simulink model "Sine_Saturation_Block"  (R2022a)
settings: Solver=VariableStepAuto  StartTime=0.0  StopTime=20  RelTol=1e-3
undefined symbols (not defined in the file or in its folder): canChannel
libraries: canlib x4, canmsglib x2
settings Model: Creator=maxju  LastModifiedBy=maxju

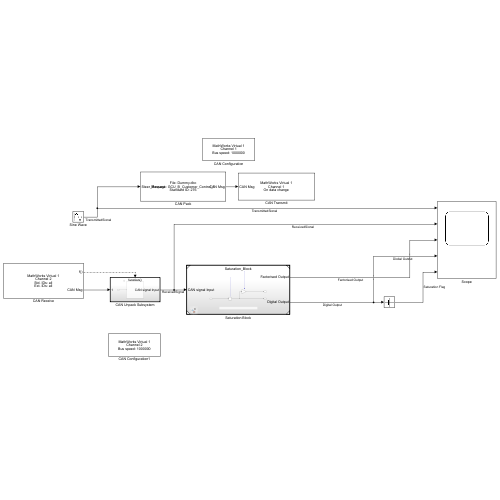
[thumbnail: Simulink's stored preview of the top-level diagram]
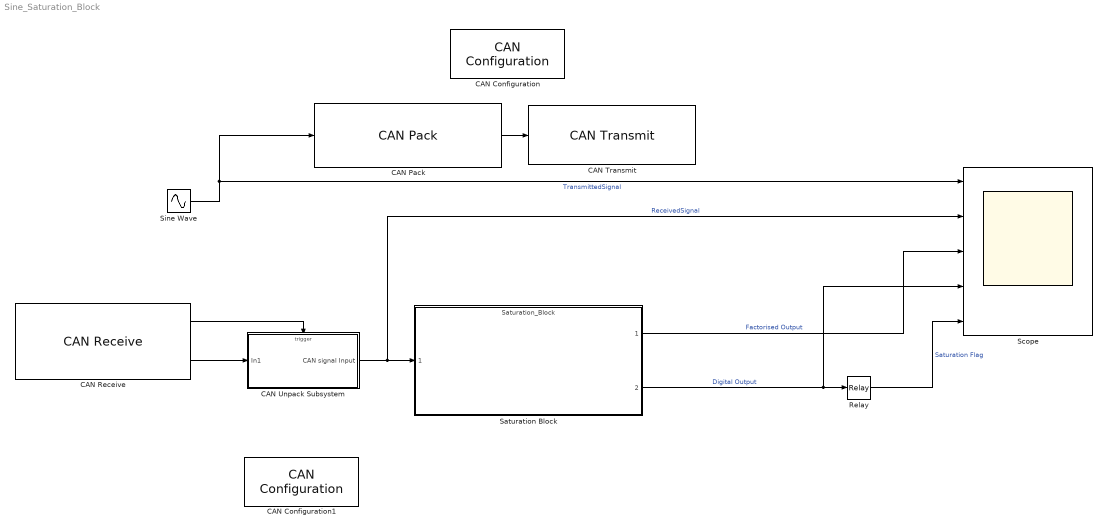
== system Sine_Saturation_Block ==
  CAN Configuration : canlib/CAN Configuration  BlockHandle=2.0009  Device=MathWorks Virtual 1 (Channel 1)  DeviceMenu=MathWorks Virtual 1 (Channel 1)  ObjConstructor=canChannel('MathWorks', 'Virtual 1', 1)  BusSpeed=1000000  EnableBitParameters=off  AckMode=Normal
      settings: SourceProductBaseCode=VN
  CAN Configuration1 : canlib/CAN Configuration  BlockHandle=3.0004  Device=MathWorks Virtual 1 (Channel 2)  DeviceMenu=MathWorks Virtual 1 (Channel 2)  ObjConstructor=canChannel('MathWorks', 'Virtual 1', 2)  BusSpeed=1000000  EnableBitParameters=off  AckMode=Normal
      settings: SourceProductBaseCode=VN
  CAN Pack : canmsglib/CAN Pack  CANdbFile=C:\Workspace\SIMULINK-Models\CAN_Saturation_Block\Dummy.dbc  MsgList=GCU_B_Customer_Control_1  MsgName=GCU_B_Customer_Control_1  MsgIDType=Standard (11-bit identifier)  MsgIdentifier=276  MsgLength=8  Remote=off  ApplyMinMax=off  BusOutput=off  SignalInfo={'Steer_Request','56','64','BE','signed','Standard','0','1','0','-100','100'}
      settings: SourceProductBaseCode=XP,ME,VN  DataFormat=CANdb specified signals
  CAN Receive : canlib/CAN Receive  BlockHandle=7.0004  Device=MathWorks Virtual 1 (Channel 2)  DeviceMenu=MathWorks Virtual 1 (Channel 2)  ObjConstructor=canChannel('MathWorks', 'Virtual 1', 2)  EnableStandardIDsFilter=off  StdIDsCombo=Allow all  StandardIDs=0  EnableExtendedIDsFilter=off  ExtIDsCombo=Allow all  ExtendedIDs=0  SampleTime=0.01  MsgsPerTimestep=1  InternalFilterUpdateStatus=on  BusOutput=off
      settings: SourceProductBaseCode=VN
  CAN Transmit : canlib/CAN Transmit  BlockHandle=10.0004  Device=MathWorks Virtual 1 (Channel 1)  DeviceMenu=MathWorks Virtual 1 (Channel 1)  ObjConstructor=canChannel('MathWorks', 'Virtual 1', 1)  EnableEventTransmit=on  EnablePeriodicTransmit=off  MessagePeriod=1.000
      settings: SourceProductBaseCode=VN
  CAN Unpack Subsystem : Subsystem  TreatAsAtomicUnit=on
  Relay : Relay  OnSwitchValue=[100 -100]  OffSwitchValue=[100 -100]  OnOutputValue=130
  Saturation Block : ModelReference  ModelNameDialog=Saturation_Block.slx  SimulationMode=Normal  ModelReferenceVersion=1.5
  Scope : Scope  NumInputPorts=5
  Sine Wave : Sin  SineType=Sample based  Amplitude=114  Samples=100  SampleTime=0.01
  wires:
  CAN Pack/1 -> CAN Transmit/1
  Sine Wave/1 -> CAN Pack/1, Scope/1  "TransmittedSignal"
  CAN Receive/2 -> CAN Unpack Subsystem/1(In1)
  CAN Receive/1 -> CAN Unpack Subsystem/Trigger
  Saturation Block/1 -> Scope/3  "Factorised Output"
  Saturation Block/2 -> Relay/1, Scope/4  "Digital Output"
  CAN Unpack Subsystem/1(CAN signal Input) -> Scope/2, Saturation Block/1  "ReceivedSignal"
  Relay/1 -> Scope/5  "Saturation Flag"

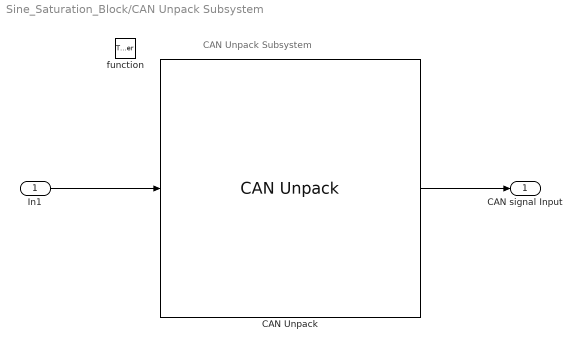
== system Sine_Saturation_Block/CAN Unpack Subsystem ==
  note: CAN Unpack Subsystem
  In1 : Inport
  function : TriggerPort  TriggerType=function-call  VariantControl=Variant
  CAN Unpack : canmsglib/CAN Unpack  CANdbFile=C:\Workspace\SIMULINK-Models\CAN_Saturation_Block\Dummy.dbc  MsgList=GCU_B_Customer_Control_1  MsgName=GCU_B_Customer_Control_1  MsgIDType=Standard (11-bit identifier)  MsgIdentifier=276  MsgLength=8  SignalInfo={'Steer_Request','56','64','BE','signed','Standard','0','1','0','-100','100'}  IDPort=off  TimestampPort=off  ErrorPort=off  RemotePort=off  LengthPort=off  StatusPort=off  ApplyMinMax=off
      settings: SourceProductBaseCode=XP,ME,VN  DataFormat=CANdb specified signals
  CAN signal Input : Outport  VectorParamsAs1DForOutWhenUnconnected=off
  wires:
  In1/1 -> CAN Unpack/1
  CAN Unpack/1 -> CAN signal Input/1
